simulink model "EcoSIM3_P2_C2"  (R2014b)
settings: Solver=ode1  SolverMode=SingleTasking  StartTime=0.0  StopTime=inf  FixedStep=0.01  RelTol=1e-3
PostLoadFcn:
  | %, if any(exist('dsrtsu_mdlpostloadfcn', 'file') == [2, 3, 6]), try dsrtsu_mdlpostloadfcn('Execute', bdroot); catch fprintf('Error in PostLoadFcn (dsrtsu_mdlpostloadfcn) for model "%s":\n %s\n', bdroot, lasterr); end, end,
InitFcn:
  | tic
  | %Startup_EcoSIM
undefined symbols (not defined in the file or in its folder): canChannel, Controls, DriveCycles, Driver, EM_EFF_MAP, EM_PwrLoss_MAP, EngPwr, EngSpd, EngTrq, Glbl, Plants, Power, Torque, Veh_Dynamics
libraries: canmsglib x100, canlib x87, fl_lib x78, simulink x59, nesl_utility x40, sdl_lib x17, dspsigops x5, dspswit3 x3, dspstat3 x2, commnoisgen2 x1, dspfdesign x1
(part 3 of 15)

== system EcoSIM3_P2_C2/Powertrain/Mechanical Coupler/Sensors ==
  note: Sensor Model: Place where we add Corrupter
  Ideal Rotational Motion Sensor : fl_lib/Mechanical/Mechanical Sensors/Ideal Rotational Motion Sensor  offset=0 rad
  Ideal Torque Sensor : fl_lib/Mechanical/Mechanical Sensors/Ideal Torque Sensor
  Mechanical Rotational Reference1 : fl_lib/Mechanical/Rotational Elements/Mechanical Rotational Reference
  PS-Simulink Converter : nesl_utility/PS-Simulink Converter  PhysicalDomain=network_engine_domain  SubClassName=ps_output  LeftPortType=input  RightPortType=output  PseudoPeriodic=off  Frequencies=[]  Unit=rad/s  AffineConversion=off
  PS-Simulink Converter1 : nesl_utility/PS-Simulink Converter  PhysicalDomain=network_engine_domain  SubClassName=ps_output  LeftPortType=input  RightPortType=output  PseudoPeriodic=off  Frequencies=[]  Unit=N*m  AffineConversion=off
  Terminator : Terminator
  Terminator1 : Terminator
  Shaft : PMIOPort  Port=1  Side=Left
  To_Plants : PMIOPort  Port=2  Side=Right
  wires:
  PS-Simulink Converter/1 -> Terminator/1  "MC_Speed_rad_per_s"
  PS-Simulink Converter1/1 -> Terminator1/1  "MC_Torque_Out_Nm"
  connections:
  Ideal Torque Sensor/LConn1 -- Shaft/RConn1 -- Ideal Rotational Motion Sensor/LConn1
  Ideal Rotational Motion Sensor/RConn1 -- Mechanical Rotational Reference1/LConn1
  PS-Simulink Converter/LConn1 -- Ideal Rotational Motion Sensor/RConn2
  PS-Simulink Converter1/LConn1 -- Ideal Torque Sensor/RConn2
  Ideal Torque Sensor/RConn1 -- To_Plants/RConn1

== system EcoSIM3_P2_C2/Powertrain/Soft_ECUs_IO/From_Goto ==
  Bus Creator : BusCreator  Inputs=7
  Subsystem : Subsystem
  Subsystem1 : Subsystem
  Supervisory_Wakeup_Terminated : Terminator
  tag scope: BAS_SoftECU_Receive=global, Brusa_SoftECU_Receive=global, Clutch_Trans_SoftECU_Receive=global, EM_SoftECU_Receive=global, ESS_SoftECU_Receive=global, Engine_SoftECU_Receive=global, From_ECUs=global, Supervisory_Receive=global
  wires:
  [ESS_SoftECU_Transmit] -> Bus Creator/1
  [EM_SoftECU_Transmit] -> Bus Creator/2
  [BAS_SoftECU_Transmit] -> Bus Creator/3
  [Engine_SoftECU_Transmit] -> Bus Creator/4
  Bus Creator/1 -> [From_ECUs]
  [GM_Transmit] -> Bus Creator/6
  [Clutch_Trans_SoftECU_Transmit] -> Bus Creator/5
  [From_Supervisory] -> Subsystem/1(Supervisory)
  Subsystem/1(ESS) -> [ESS_SoftECU_Receive]
  Subsystem/2(EM) -> [EM_SoftECU_Receive]
  Subsystem/3(BAS) -> [BAS_SoftECU_Receive]
  Subsystem/4(ICE) -> [Engine_SoftECU_Receive]
  Subsystem/5(Trans) -> [Clutch_Trans_SoftECU_Receive]
  Subsystem/6(Super) -> [Supervisory_Receive]
  [From_GCM] -> Subsystem1/1(From_GCM)
  Subsystem1/1(SoftECUPowerup) -> Subsystem/2(Relay Powerups)
  Subsystem1/2(MABxPowerup) -> Supervisory_Wakeup_Terminated/1
  Subsystem/7(Brusa) -> [Brusa_SoftECU_Receive]
  [Brusa_SoftECU_Transmit] -> Bus Creator/7

== system EcoSIM3_P2_C2/Powertrain/Soft_ECUs_IO/VNT Kvaser ==
  CANRx : Subsystem
  CANTx : Subsystem
  ElectricalRx : Subsystem
  ElectricalTx : Subsystem
  Spine : Subsystem
  wires:
  ElectricalRx/1(Electrical) -> Spine/1(Electrical)
  CANRx/1(CAN Out) -> Spine/2(CAN)
  Spine/1(ElectricalTx) -> ElectricalTx/1(Electrical)
  Spine/2(CANTx) -> CANTx/1(CAN)

== system EcoSIM3_P2_C2/Powertrain/Soft_ECUs_IO/VNT Vector ==
  CANRx : Subsystem
  CANTx : Subsystem
  ElectricalRx : Subsystem
  ElectricalTx : Subsystem
  Spine : Subsystem
  wires:
  ElectricalRx/1(Electrical) -> Spine/1(Electrical)
  CANRx/1(CAN Out) -> Spine/2(CAN)
  Spine/1(ElectricalTx) -> ElectricalTx/1(Electrical)
  Spine/2(CANTx) -> CANTx/1(CAN)

== system EcoSIM3_P2_C2/Powertrain/Vehicle Dynamics/Sensor ==
  Bus Creator : BusCreator  Inputs=5
  Ideal Rotational Motion Sensor{,1..3} (4 alike) : fl_lib/Mechanical/Mechanical Sensors/Ideal Rotational Motion Sensor  offset=0 rad
  Mechanical Rotational Reference{,1..3} (4 alike) : fl_lib/Mechanical/Rotational Elements/Mechanical Rotational Reference
  PS-Simulink Converter{1..2,4..5} (4 alike) : nesl_utility/PS-Simulink Converter  PhysicalDomain=network_engine_domain  SubClassName=ps_output  LeftPortType=input  RightPortType=output  PseudoPeriodic=off  Frequencies=[]  Unit=rad  AffineConversion=off
  PS-Simulink Converter3 : nesl_utility/PS-Simulink Converter  PhysicalDomain=network_engine_domain  SubClassName=ps_output  LeftPortType=input  RightPortType=output  PseudoPeriodic=off  Frequencies=[]  Unit=m/s  AffineConversion=off
  Sensor lag : Subsystem
  Sensor lag1 : Subsystem
  Sensor lag2 : Subsystem
  Sensor lag3 : Subsystem
  Sensor lag4 : Subsystem
  Vehicle_Speed : PMIOPort  Port=1  Side=Left
  FLT : PMIOPort  Port=2  Side=Left
  FRT : PMIOPort  Port=3  Side=Left
  RLT : PMIOPort  Port=4  Side=Right
  RRT : PMIOPort  Port=5  Side=Right
  Sensor_Out : Outport
  wires:
  PS-Simulink Converter3/1 -> Sensor lag/1(i)
  Sensor lag/1(o) -> Bus Creator/1  "Vehicle_Speed_meter_per_s"
  PS-Simulink Converter1/1 -> Sensor lag1/1(i)
  PS-Simulink Converter2/1 -> Sensor lag2/1(i)
  PS-Simulink Converter4/1 -> Sensor lag3/1(i)
  PS-Simulink Converter5/1 -> Sensor lag4/1(i)
  Sensor lag1/1(o) -> Bus Creator/2  "Front_Left_Tire_Angle"
  Sensor lag3/1(o) -> Bus Creator/3  "Rear_Left_Tire_Angle"
  Sensor lag2/1(o) -> Bus Creator/4  "Front_Right_Tire_Angle"
  Sensor lag4/1(o) -> Bus Creator/5  "Rear_Right_Tire_Angle"
  Bus Creator/1 -> Sensor_Out/1
  connections:
  Vehicle_Speed/RConn1 -- PS-Simulink Converter3/LConn1
  Ideal Rotational Motion Sensor/LConn1 -- FLT/RConn1
  Ideal Rotational Motion Sensor1/LConn1 -- FRT/RConn1
  Ideal Rotational Motion Sensor/RConn1 -- Mechanical Rotational Reference/LConn1
  Ideal Rotational Motion Sensor2/RConn1 -- Mechanical Rotational Reference1/LConn1
  Ideal Rotational Motion Sensor3/RConn1 -- Mechanical Rotational Reference2/LConn1
  Ideal Rotational Motion Sensor1/RConn1 -- Mechanical Rotational Reference3/LConn1
  PS-Simulink Converter1/LConn1 -- Ideal Rotational Motion Sensor/RConn3
  PS-Simulink Converter2/LConn1 -- Ideal Rotational Motion Sensor1/RConn3
  Ideal Rotational Motion Sensor2/RConn3 -- PS-Simulink Converter4/LConn1
  PS-Simulink Converter5/LConn1 -- Ideal Rotational Motion Sensor3/RConn3
  RRT/RConn1 -- Ideal Rotational Motion Sensor3/LConn1
  RLT/RConn1 -- Ideal Rotational Motion Sensor2/LConn1

== system EcoSIM3_P2_C2/Powertrain/Vehicle Dynamics/Subsystem ==
  Ideal Force Sensor : fl_lib/Mechanical/Mechanical Sensors/Ideal Force Sensor
  R : PMIOPort  Port=1  Side=Right
  C : PMIOPort  Port=2  Side=Left
  F : PMIOPort  Port=3  Side=Left
  connections:
  Ideal Force Sensor/LConn1 -- R/RConn1
  Ideal Force Sensor/RConn1 -- C/RConn1
  F/RConn1 -- Ideal Force Sensor/RConn2

== system EcoSIM3_P2_C2/RTI Data/RTI Data Store/RTI Data Store ==
  RTI Data Store : Subsystem  mask(RTI_DATA_STORE){}
      mask help:
      | RTI Data Store Block. This block is used by RTI to store internal model dependent data. Deleting this block will result in data loss.
      |
      | NEVER DELETE, COPY, OR MODIFY THIS BLOCK!
      mask Help:
      | RTI Data Store Block. This block is used by RTI to store internal model dependent data. Deleting this block will result in data loss.
      | 
      | NEVER DELETE, COPY, OR MODIFY THIS BLOCK!
      mask Display: text(0.5, 0.5, ' ', 'HorizontalAlignment', 'center');

== system EcoSIM3_P2_C2/Supervisory Controller/Driver Requested Torque/Max Torque Calculation ==
  note: at the wheels
  Gear : Inport
  Engine Speed : Inport  Port=2
  Divide2 : Product  Inputs=**
  Max Torque : Lookup_n-D  NumberOfTableDimensions=1  BreakpointsForDimension1=Plants.ICE.Mdl.Plant.Max_Trq.w  Table=Plants.ICE.Mdl.Plant.Max_Trq.Trq  InternalRulePriority=Speed  RndMeth=Simplest  InputSameDT=on
  RearGR3 : Gain  Gain=2.77
  TRAN GR2 : Lookup_n-D  NumberOfTableDimensions=1  BreakpointsForDimension1=Plants.Trans.Mdl.Plant.Gear_cmd  Table=Plants.Trans.Mdl.Plant.GR  ExtrapMethod=Clip  InternalRulePriority=Speed  RndMeth=Simplest  InputSameDT=on
  "Engine Torque " : Outport
  wires:
  TRAN GR2/1 -> Divide2/2
  Gear/1 -> TRAN GR2/1
  Engine Speed/1 -> Max Torque/1
  Divide2/1 -> "Engine Torque "/1
  Max Torque/1 -> RearGR3/1  "Engine Torque"
  RearGR3/1 -> Divide2/1

== system EcoSIM3_P2_C2/Supervisory Controller/Driver Requested Torque/Speed Calculations ==
  "Vehicle Speed m/s " : Inport
  Gear Current : Inport  Port=2
  Gain1 : Gain  Gain=2/Plants.Rear_wh.tire_diameter
  Gain2 : Gain  Gain=2.77
  Product : Product
  TRAN GR : Lookup_n-D  NumberOfTableDimensions=1  BreakpointsForDimension1=Plants.Trans.Mdl.Plant.Gear_cmd  Table=Plants.Trans.Mdl.Plant.GR  ExtrapMethod=Clip  InternalRulePriority=Speed  RndMeth=Simplest  InputSameDT=on
  Engine Speed : Outport
  "EM Speed " : Outport  Port=2
  wires:
  "Vehicle Speed m/s "/1 -> Gain1/1
  Gain2/1 -> "EM Speed "/1, Product/2
  Gain1/1 -> Gain2/1
  Product/1 -> Engine Speed/1
  Gear Current/1 -> TRAN GR/1
  TRAN GR/1 -> Product/1

== system EcoSIM3_P2_C2/Supervisory Controller/Functional Safety1/Functional Safety Algorithm ==
  Torque Requests : Inport
  ECU/Sensor Signals : Inport  Port=2
  Fault Detection (Team Developed) : Subsystem
  Fault Management : Subsystem
  Fault Mitigation : Subsystem
  Torque Limits : Outport
  Fault Code : Outport  Port=2
  wires:
  Torque Requests/1 -> Fault Detection (Team Developed)/1(Torque Requests)
  ECU/Sensor Signals/1 -> Fault Detection (Team Developed)/2(ECU/Sensor Signals), Fault Management/2(ECU/Sensor Signals)
  Fault Mitigation/1(Torque Limits) -> Torque Limits/1
  Fault Management/1(Fault Code) -> Fault Mitigation/1(Fault Code), Fault Code/1
  Fault Detection (Team Developed)/1(Team Dev Fault Signals) -> Fault Management/1(Team Dev Fault Signals)

== system EcoSIM3_P2_C2/Supervisory Controller/Input Conditioning/Alpha Conditioning ==
  Raw Alpha_V : Inport
  Add : Sum
  Bus Selector : BusSelector  OutputSignals=GM_Transmit.GM_Electrical_Out.Alpha_Low,GM_Transmit.GM_Electrical_Out.Alpha_High
  Constant : Constant  Value=0.4
  Constant1 : Constant  Value=0.8
  Output Scaling5 : Gain  Gain=50
  Output Scaling6 : Gain  Gain=25
  Output Scaling7 : Gain  Gain=0.5
  Sum4 : Sum  Inputs=-+|
  Sum5 : Sum  Inputs=|+-
  Alpha Percent : Outport
  wires:
  Constant1/1 -> Sum5/2
  Sum5/1 -> Output Scaling6/1
  Output Scaling5/1 -> Add/1
  Output Scaling7/1 -> Alpha Percent/1  "Alpha_percent"
  Bus Selector/1 -> Sum4/2  "<Alpha_Low>"
  Output Scaling6/1 -> Add/2
  Constant/1 -> Sum4/1
  Add/1 -> Output Scaling7/1
  Sum4/1 -> Output Scaling5/1
  Bus Selector/2 -> Sum5/1  "<Alpha_High>"
  Raw Alpha_V/1 -> Bus Selector/1

== system EcoSIM3_P2_C2/Supervisory Controller/Input Conditioning/Velocity Conditioning ==
  Raw Ticks : Inport
  Bus Creator : BusCreator  Inputs=2
  Bus Selector1 : BusSelector  OutputSignals=GM_Transmit.GMLAN_CAN_Out.PPEI_Vehicle_Speed_and_Distance.VehSpdAvgDrvn,GM_Transmit.GMLAN_CAN_Out.PPEI_Driven_Whl_Rotational_Stat.WRSLDWhlDistPlsCntr,GM_Transmit.GMLAN_CAN_Out.PPEI_Driven_Whl_Rotational_Stat.WRSRDWhlDistPlsCntr,GM_Transmit.GMLAN_CAN_Out.PPEI_NonDrivn_Whl_Rotationl_Stat.WRSLNDWhlDistPCntr,GM_Transmit.GMLAN_CAN_Out.PPEI_NonDrivn_Whl_Rotationl_Stat.WRSRNDWhlDistPCntr
  Gain : Gain  Gain=1/3.6
  Mean : dspstat3/Mean  run=off  reset_popup=None  InputProcessing=Columns as channels (frame based)  directionMode=Each column  dimension=1  treatSBRowAsCol=on  roiEnable=off  roiType=Rectangles  roiPortion=Entire ROI  roiOutput=Individual statistics for each ROI  roiFlag=off  outputDataTypeStr=Inherit: Same as accumulator  outputLastDataTypeStr=Inherit: Same as accumulator  outputMin=[]  outputMax=[]  roundingMode=Floor  overflowMode=off
  Mux : Mux
  Subsystem : Subsystem
  Subsystem1 : Subsystem
  Subsystem2 : Subsystem
  Subsystem3 : Subsystem
  Velocity Processed : Outport
  wires:
  Bus Selector1/5 -> Subsystem3/1(In1)  "<WRSRNDWhlDistPCntr>"
  Bus Selector1/4 -> Subsystem2/1(In1)  "<WRSLNDWhlDistPCntr>"
  Raw Ticks/1 -> Bus Selector1/1
  Bus Selector1/1 -> Gain/1  "<VehSpdAvgDrvn>"
  Bus Selector1/3 -> Subsystem1/1(In1)  "<WRSRDWhlDistPlsCntr>"
  Bus Creator/1 -> Velocity Processed/1  "Vehicle_speed"
  Mean/1 -> Bus Creator/2  "Processed_Speed_m_per_sec"
  Gain/1 -> Bus Creator/1  "Vehicle_Speed_meter_per_s"
  Bus Selector1/2 -> Subsystem/1(In1)  "<WRSLDWhlDistPlsCntr>"
  Subsystem2/1(Speed_LND) -> Mux/3
  Subsystem1/1(Speed_RD) -> Mux/2
  Subsystem/1(Speed_LD) -> Mux/1
  Subsystem3/1(Speed_RND) -> Mux/4
  Mux/1 -> Mean/1

== system EcoSIM3_P2_C2/Supervisory Controller/Mode Operation/Accessory ==
  "Supervisory " : Inport
  Enable : EnablePort  StatesWhenEnabling=reset
  BAS_Signals : Subsystem
  Bus Creator2 : BusCreator  Inputs=8
  Constant1 : Constant  Value=0
  DC/DC Enabled : Subsystem
  ESS_Messages : Subsystem
  Engine Messages : Subsystem
  Signal Conversion : SignalConversion
  TM Messages : Subsystem
  Trans_Messages : Subsystem
  Output : Outport
  wires:
  Signal Conversion/1 -> Output/1  "HSC_Output"
  Engine Messages/1(Out1) -> Bus Creator2/5
  ESS_Messages/1(Out1) -> Bus Creator2/2  "ESS_Signals_A123"
  Trans_Messages/1(Out1) -> Bus Creator2/6  "Trans_Receive"
  BAS_Signals/1(Out1) -> Bus Creator2/4  "BAS_SoftECU_Receive"
  "Supervisory "/1 -> Bus Creator2/7  "Supervisory"
  Bus Creator2/1 -> Signal Conversion/1  "HSC_Output"
  DC/DC Enabled/1(Out1) -> Bus Creator2/8
  TM Messages/1(Out1) -> Bus Creator2/3
  Constant1/1 -> Bus Creator2/1  "Vehicle_Ready"

== system EcoSIM3_P2_C2/Supervisory Controller/Mode Operation/Charging ==
  From CAN : Inport
  "Supervisory " : Inport  Port=2
  Enable : EnablePort  StatesWhenEnabling=reset
  BAS_Signals : Subsystem
  Bus Creator2 : BusCreator  Inputs=8
  Constant2 : Constant  Value=0
  DC/DC Enabled : Subsystem
  EM_Signals : Subsystem
  ESS_Messages : Subsystem
  Engine Messages : Subsystem
  Signal Conversion : SignalConversion
  Trans_Messages : Subsystem
  Output : Outport
  wires:
  Signal Conversion/1 -> Output/1  "HSC_Output"
  Engine Messages/1(Out1) -> Bus Creator2/5
  ESS_Messages/1(Out1) -> Bus Creator2/2  "ESS_Signals_A123"
  Trans_Messages/1(Out1) -> Bus Creator2/6  "Trans_Receive"
  BAS_Signals/1(Out1) -> Bus Creator2/4  "BAS_SoftECU_Receive"
  From CAN/1 -> ESS_Messages/1(From CAN)
  "Supervisory "/1 -> Bus Creator2/7  "Supervisory"
  Bus Creator2/1 -> Signal Conversion/1  "HSC_Output"
  EM_Signals/1(Out1) -> Bus Creator2/3
  DC/DC Enabled/1(Out1) -> Bus Creator2/8
  Constant2/1 -> Bus Creator2/1  "Vehicle_Ready"

== system EcoSIM3_P2_C2/Supervisory Controller/Mode Operation/EV ==
  "Supervisory " : Inport
  CAN : Inport  Port=2
  Enable : EnablePort  StatesWhenEnabling=reset
  BAS_Signals : Subsystem
  Bus Creator1 : BusCreator  Inputs=8
  Bus Creator2 : BusCreator  Inputs=3
  Bus Selector : BusSelector  OutputSignals=Driver Torque Request
  Bus Selector1 : BusSelector  OutputSignals=EM_Transmit.EM_CAN_Out.M165_Motor_Position_Info.Motor_Speed,EM_Transmit.EM_CAN_Out.M162_Temperature_Set_3.Motor_Temperature
  Constant1 : Constant  Value=0
  Constant2 : Constant
  Constant4 : Constant
  Constant5 : Constant  Value=0
  DC/DC Enabled : Subsystem
  EM Max Torque1 : Lookup_n-D  NumberOfTableDimensions=1  BreakpointsForDimension1=Plants.EM.Mdl.Plant.max_min_RPM  BreakpointsForDimension2=[25,70]  Table=[Plants.EM.Mdl.Plant.T_max_Peak]  InternalRulePriority=Speed  RndMeth=Simplest  InputSameDT=on
  ESS_Messages : Subsystem
  Engine Messages : Subsystem
  Gain : Gain  Gain=1/(2.77*2.77)
  Saturation Dynamic : simulink/Discontinuities/Saturation Dynamic  OutMin=[]  OutMax=[]  OutDataTypeStr=Inherit: Same as second input  OutDataType=fixdt(1, 16)  OutScaling=2^-10  DoSatur=off
  Signal Conversion : SignalConversion
  Trans_Messages : Subsystem
  Output : Outport
  wires:
  Signal Conversion/1 -> Output/1  "HSC_Output"
  Engine Messages/1(Out1) -> Bus Creator1/5
  ESS_Messages/1(Out1) -> Bus Creator1/2  "ESS_Signals_A123"
  Bus Creator2/1 -> Bus Creator1/3  "EM_Messages_Rhinehart"
  Gain/1 -> Saturation Dynamic/2  "Torque_Command"
  Constant1/1 -> Bus Creator2/3  "Rotation_Direction"
  Constant2/1 -> Bus Creator2/1  "Inverter_Enable"
  Trans_Messages/1(Out1) -> Bus Creator1/6  "Trans_Receive"
  BAS_Signals/1(Out1) -> Bus Creator1/4  "BAS_SoftECU_Receive"
  "Supervisory "/1 -> Bus Creator1/7, Bus Selector/1  "Supervisory"
  Bus Creator1/1 -> Signal Conversion/1  "HSC_Output"
  Bus Selector/1 -> Gain/1  "<Driver Torque Request>"
  Constant4/1 -> Bus Creator1/1  "Vehicle_Ready"
  DC/DC Enabled/1(Out1) -> Bus Creator1/8
  Saturation Dynamic/1 -> Bus Creator2/2  "Torque_Command"
  Constant5/1 -> Saturation Dynamic/3
  CAN/1 -> Bus Selector1/1
  Bus Selector1/1 -> EM Max Torque1/1  "<Motor_Speed>"
  Bus Selector1/2 -> ?  "<Motor_Temperature>"
  EM Max Torque1/1 -> Saturation Dynamic/1

== system EcoSIM3_P2_C2/Supervisory Controller/Mode Operation/Engine Only  ==
  note: this will end up being engine idle in the vehicle
  "Supervisory " : Inport
  From CAN : Inport  Port=2
  Enable : EnablePort  StatesWhenEnabling=reset
  BAS_Signals : Subsystem
  Bus Creator1 : BusCreator  Inputs=8
  Bus Creator6 : BusCreator  Inputs=2
  Constant1 : Constant
  Constant2 : Constant  Value=0
  Constant4 : Constant
  DC/DC Enabled : Subsystem
  ESS_Messages : Subsystem
  Engine Messages : Subsystem
  Signal Conversion : SignalConversion
  Subsystem : Subsystem
  Supervisory 1 : InportShadow
  TM Messages : Subsystem
  Terminator : Terminator
  Terminator1 : Terminator
  "Output " : Outport
  wires:
  Signal Conversion/1 -> "Output "/1  "HSC_Output"
  ESS_Messages/1(Out1) -> Bus Creator1/2  "ESS_Signals_A123"
  Bus Creator6/1 -> Bus Creator1/6  "Trans_Receive"
  BAS_Signals/1(Out1) -> Bus Creator1/4  "BAS_SoftECU_Receive"
  Constant2/1 -> Bus Creator6/1  "Shift_Request"
  Subsystem/3("Gear Requested ") -> Terminator1/1  "Gear_Request"
  "Supervisory "/1 -> Bus Creator1/7, Subsystem/2(Supervisory)  "Supervisory"
  Bus Creator1/1 -> Signal Conversion/1  "HSC_Output"
  From CAN/1 -> Subsystem/1(From CAN)
  Subsystem/2(Shift Requested) -> Terminator/1
  Constant1/1 -> Bus Creator6/2  "Gear_Request"
  Constant4/1 -> Bus Creator1/1  "Vehicle_Ready"
  DC/DC Enabled/1(Out1) -> Bus Creator1/8
  TM Messages/1(Out1) -> Bus Creator1/3
  Engine Messages/1(Out1) -> Bus Creator1/5
  Supervisory 1/1 -> TM Messages/1(In1)  "Supervisory"

== system EcoSIM3_P2_C2/Supervisory Controller/Mode Operation/Engine Start  ==
  "Supervisory " : Inport
  "CAN In " : Inport  Port=2
  Enable : EnablePort  StatesWhenEnabling=reset
  1-D Lookup Table : Lookup_n-D  NumberOfTableDimensions=1  BreakpointsForDimension1=[0 2699 2700 3000 3239 3240]  Table=[11.11 11.11 8 5.5 5.5 0]  InternalRulePriority=Speed  RndMeth=Simplest  InputSameDT=on
  Bus Creator1 : BusCreator  Inputs=8
  Bus Creator2 : BusCreator  Inputs=3
  Bus Creator4 : BusCreator  Inputs=3
  Bus Selector : BusSelector  OutputSignals=BAS_Transmit.BAS_CAN_Out.Status_1.BAS_Speed_rad_per_s
  Compare To Constant : simulink/Logic and Bit Operations/Compare To Constant  relop=>  const=900  OutDataTypeStr=boolean
  Constant1 : Constant  Value=0
  Constant3 : Constant  Value=0
  Constant4 : Constant
  Constant5 : Constant
  Constant6 : Constant
  Convert to Engine Speed : Gain  Gain=1/2.7
  DC/DC Enabled : Subsystem
  Data Type Conversion : DataTypeConversion  OutDataTypeStr=double
  ESS_Messages : Subsystem
  Sample and Hold : dspsigops/Sample and Hold  trig=Rising edge  initCond=0  latchinput=off
  Signal Conversion : SignalConversion
  Supervisory 1 : InportShadow
  TM Messages : Subsystem
  Trans Messages : Subsystem
  rad/sec to RPM : Gain  Gain=9.54929659643
  rad/sec to RPM1 : Gain  Gain=1.1
  "Output " : Outport
  wires:
  Signal Conversion/1 -> "Output "/1  "HSC_Output"
  ESS_Messages/1(Out1) -> Bus Creator1/2  "ESS_Signals_A123"
  "Supervisory "/1 -> Bus Creator1/7  "Supervisory"
  Bus Creator1/1 -> Signal Conversion/1  "HSC_Output"
  Constant5/1 -> Bus Creator1/1  "Vehicle_Ready"
  DC/DC Enabled/1(Out1) -> Bus Creator1/8
  TM Messages/1(Out1) -> Bus Creator1/3
  Constant6/1 -> Bus Creator4/3  "BAS_Mode_Request"
  Bus Creator4/1 -> Bus Creator1/4  "BAS_SoftECU_Receive"
  Trans Messages/1(Out1) -> Bus Creator1/6
  Supervisory 1/1 -> TM Messages/1(In1)  "Supervisory"
  Constant3/1 -> Bus Creator2/1  "ICE_Torque_Request_Nm"
  1-D Lookup Table/1 -> rad/sec to RPM1/1  "BAS_Torque_Request_Nm"
  Constant1/1 -> Bus Creator4/2  "BAS_Speed_Request"
  Constant4/1 -> Bus Creator2/2  "Engine_On"
  "CAN In "/1 -> Bus Selector/1
  Bus Selector/1 -> rad/sec to RPM/1  "<BAS_Speed_rad_per_s>"
  rad/sec to RPM/1 -> Convert to Engine Speed/1, 1-D Lookup Table/1  "BAS_Speed_RPM"
  Bus Creator2/1 -> Bus Creator1/5  "ICE_Request"
  Compare To Constant/1 -> Data Type Conversion/1
  Convert to Engine Speed/1 -> Compare To Constant/1
  Data Type Conversion/1 -> Sample and Hold/Trigger, Sample and Hold/1  "Engine_Run"
  Sample and Hold/1 -> Bus Creator2/3  "Engine_Run"
  rad/sec to RPM1/1 -> Bus Creator4/1  "BAS_Torque_Request_Nm"

== system EcoSIM3_P2_C2/Supervisory Controller/Mode Operation/Limited EV ==
  "Supervisory " : Inport
  CAN : Inport  Port=2
  Enable : EnablePort  StatesWhenEnabling=reset
  BAS_Signals : Subsystem
  Bus Creator3 : BusCreator  Inputs=8
  Bus Creator4 : BusCreator  Inputs=3
  Bus Selector : BusSelector  OutputSignals=Driver Torque Request
  Bus Selector1 : BusSelector  OutputSignals=EM_Transmit.EM_CAN_Out.M162_Temperature_Set_3.Motor_Temperature,ESS_Transmit.ESS_CAN_Out.BCM_Data1.bcm_cell_tmax,EM_Transmit
  Constant1 : Constant
  Constant2 : Constant  Value=0
  Constant4 : Constant
  DC/DC Enabled : Subsystem
  ESS_Messages : Subsystem
  Engine Messages : Subsystem
  Gain1 : Gain  Gain=1/(2.77*2.77)
  "Inverter Temp Selection " : Subsystem
  Signal Conversion : SignalConversion
  Temperature Limiting : Subsystem
  Trans_Messages : Subsystem
  Output : Outport
  wires:
  Signal Conversion/1 -> Output/1  "HSC_Output"
  ESS_Messages/1(Out1) -> Bus Creator3/2  "ESS_Signals_A123"
  Bus Creator4/1 -> Bus Creator3/3  "EM_Messages_Rhinehart"
  Bus Selector/1 -> Gain1/1  "<Driver Torque Request>"
  Constant2/1 -> Bus Creator4/3  "Rotation_Direction"
  Constant4/1 -> Bus Creator4/1  "Inverter_Enable"
  Trans_Messages/1(Out1) -> Bus Creator3/6  "Trans_Receive"
  BAS_Signals/1(Out1) -> Bus Creator3/4  "BAS_SoftECU_Receive"
  "Supervisory "/1 -> Bus Creator3/7, Bus Selector/1  "Supervisory"
  Bus Creator3/1 -> Signal Conversion/1  "HSC_Output"
  Constant1/1 -> Bus Creator3/1  "Vehicle_Ready"
  DC/DC Enabled/1(Out1) -> Bus Creator3/8
  Gain1/1 -> Temperature Limiting/1(Torque Request)  "Torque_Command"
  Bus Selector1/1 -> Temperature Limiting/2("Motor Temperature ")  "<Motor_Temperature>"
  "Inverter Temp Selection "/1(Out1) -> Temperature Limiting/4("Inverter Temperature ")
  CAN/1 -> Bus Selector1/1
  Temperature Limiting/1(Torque Command) -> Bus Creator4/2  "Torque_Command"
  Bus Selector1/2 -> Temperature Limiting/3("Battery Temperature ")  "<bcm_cell_tmax>"
  Engine Messages/1(Out1) -> Bus Creator3/5
  Bus Selector1/3 -> "Inverter Temp Selection "/1(In1)  "<EM_Transmit>"

== system EcoSIM3_P2_C2/Supervisory Controller/Mode Operation/Series ==
  "Supervisory " : Inport
  From CAN : Inport  Port=2
  Enable : EnablePort  StatesWhenEnabling=reset
  Bus Creator1 : BusCreator  Inputs=8
  Bus Creator2 : BusCreator  Inputs=3
  Bus Creator4 : BusCreator  Inputs=3
  Bus Creator5 : BusCreator  Inputs=3
  Bus Selector : BusSelector  OutputSignals=Driver Torque Request
  Constant1 : Constant  Value=2
  Constant{2,5,7..8} (4 alike) : Constant
  Constant3 : Constant  Value=0
  Constant4 : Constant  Value=0
  DC/DC Enabled : Subsystem
  ESS_Messages : Subsystem
  Gain : Gain
  Gain1 : Gain  Gain=1/(2.77*2.77)
  "Series Torque Determination " : Subsystem
  Signal Conversion : SignalConversion
  Supervisory 1 : InportShadow
  Trans_Messages : Subsystem
  "Output " : Outport
  wires:
  Bus Creator1/1 -> Signal Conversion/1  "HSC_Output"
  "Supervisory "/1 -> Bus Creator1/7  "Supervisory"
  Bus Selector/1 -> Gain1/1  "<Driver Torque Request>"
  Supervisory 1/1 -> Bus Selector/1  "Supervisory"
  Constant5/1 -> Bus Creator5/1  "Inverter_Enable"
  Constant3/1 -> Bus Creator5/3  "Rotation_Direction"
  Bus Creator5/1 -> Bus Creator1/3  "EM_Messages_Rhinehart"
  ESS_Messages/1(Out1) -> Bus Creator1/2  "ESS_Signals_A123"
  Signal Conversion/1 -> "Output "/1  "HSC_Output"
  Trans_Messages/1(Out1) -> Bus Creator1/6  "Trans_Receive"
  Bus Creator4/1 -> Bus Creator1/4  "BAS_SoftECU_Receive"
  Constant1/1 -> Bus Creator4/3  "BAS_Mode_Request"
  DC/DC Enabled/1(Out1) -> Bus Creator1/8
  Constant2/1 -> Bus Creator1/1  "Vehicle_Ready"
  Gain1/1 -> Bus Creator5/2  "Torque_Command"
  "Series Torque Determination "/2(Engine Torque) -> Gain/1
  "Series Torque Determination "/1(BAS Speed) -> Bus Creator4/2  "BAS_Speed_Request"
  Constant4/1 -> Bus Creator4/1  "BAS_Torque_Request_Nm"
  From CAN/1 -> "Series Torque Determination "/1(Battery SOC)
  Gain/1 -> Bus Creator2/1  "ICE_Torque_Request_Nm"
  Constant7/1 -> Bus Creator2/2  "Engine_On"
  Constant8/1 -> Bus Creator2/3  "Engine_Run"
  Bus Creator2/1 -> Bus Creator1/5  "ICE_Request"

== system EcoSIM3_P2_C2/Supervisory Controller/Mode Operation/Shutdown ==
  From CAN : Inport
  "Supervisory " : Inport  Port=2
  Enable : EnablePort  StatesWhenEnabling=reset
  BAS_Signals : Subsystem
  Bus Creator2 : BusCreator  Inputs=8
  Bus Creator3 : BusCreator  Inputs=3
  Bus Selector : BusSelector  OutputSignals=EM_Transmit.EM_CAN_Out.M170_Internal_States.Inverter_Enable_Lockout
  Constant3 : Constant  Value=0
  Constant6 : Constant  Value=0
  DC/DC Disabled : Subsystem
  EM Handshake : Stateflow chart  TreatAsAtomicUnit=on
  Engine Messages : Subsystem
  Shutdown : Subsystem
  Shutdown Complete : Subsystem
  Signal Conversion : SignalConversion
  Trans_Messages : Subsystem
  Output : Outport
  wires:
  Signal Conversion/1 -> Output/1  "HSC_Output"
  Engine Messages/1(Out1) -> Bus Creator2/5
  Shutdown/1(Out1) -> Shutdown Complete/1(In1), Bus Creator2/2
  Bus Creator3/1 -> Bus Creator2/3  "EM_Messages_Rhinehart"
  Constant6/1 -> Bus Creator3/2  "Torque_Command"
  Constant3/1 -> Bus Creator3/3  "Rotation_Direction"
  EM Handshake/1(Inverter_Enable) -> Shutdown Complete/2(In2), Bus Creator3/1  "Inverter_Enable"
  Trans_Messages/1(Out1) -> Bus Creator2/6  "Trans_Receive"
  BAS_Signals/1(Out1) -> Bus Creator2/4  "BAS_SoftECU_Receive"
  From CAN/1 -> Shutdown/1(In1), Bus Selector/1
  "Supervisory "/1 -> Bus Creator2/7  "Supervisory"
  Bus Selector/1 -> EM Handshake/1(Inverter_Enable_Lockout)  "<Inverter_Enable_Lockout>"
  Bus Creator2/1 -> Signal Conversion/1  "HSC_Output"
  DC/DC Disabled/1(Out1) -> Bus Creator2/8
  Shutdown Complete/1(Out1) -> Bus Creator2/1  "Vehicle_Ready"

== system EcoSIM3_P2_C2/Supervisory Controller/Mode Operation/Startup ==
  From CAN : Inport
  "Supervisory " : Inport  Port=2
  Enable : EnablePort  StatesWhenEnabling=reset
  BAS Start up : Subsystem
  "Battery Start Up " : Subsystem
  Bus Creator1 : BusCreator  Inputs=8
  Bus Selector : BusSelector  OutputSignals=ESS_Transmit.ESS_CAN_Out.BCM_Status.bcm_mainc_stat
  Bus Selector1 : BusSelector  OutputSignals=Inverter_Enable
  Bus Selector2 : BusSelector  OutputSignals=BAS_Mode_Request
  DC/DC Enabled : Subsystem
  EM Start up : Subsystem
  Engine Messages : Subsystem
  Signal Conversion : SignalConversion
  "Start up overide " : Subsystem
  To Workspace : ToWorkspace  VariableName=StartComplete  SaveFormat=Structure With Time  SampleTime=-1
  To Workspace1 : ToWorkspace  VariableName=bcm_mainc_stat  SaveFormat=Structure With Time  SampleTime=-1
  To Workspace2 : ToWorkspace  VariableName=Inverter_enable  SaveFormat=Structure With Time  SampleTime=-1
  To Workspace3 : ToWorkspace  VariableName=BAS_Enabled  SaveFormat=Structure With Time  SampleTime=-1
  To Workspace4 : ToWorkspace  VariableName=VehReady2  SaveFormat=Structure With Time  SampleTime=-1
  Trans_Messages : Subsystem
  Vehicle Ready : Stateflow chart  TreatAsAtomicUnit=on
  "Vehicle Start Up " : Subsystem
  Output : Outport
  wires:
  Bus Creator1/1 -> Signal Conversion/1
  BAS Start up/1(Out1) -> Bus Selector2/1, Bus Creator1/4  "BAS_SoftECU_Receive"
  Trans_Messages/1(Out1) -> Bus Creator1/6  "Trans_Receive"
  "Battery Start Up "/1(Out1) -> Bus Creator1/2
  EM Start up/1(Out1) -> Bus Selector1/1, Bus Creator1/3
  Bus Selector/1 -> To Workspace1/1, Vehicle Ready/2(bcm_mainc_stat)  "<bcm_mainc_stat>"
  Bus Selector1/1 -> Vehicle Ready/3(Inverter_Enable), To Workspace2/1  "<Inverter_Enable>"
  Bus Selector2/1 -> To Workspace3/1, Vehicle Ready/4(BAS_Mode_Request)  "<BAS_Mode_Request>"
  Vehicle Ready/1(Vehicle_Ready) -> To Workspace4/1, Bus Creator1/1  "Vehicle_Ready"
  "Supervisory "/1 -> Bus Creator1/7  "Supervisory"
  Signal Conversion/1 -> Output/1  "HSC_Output"
  "Vehicle Start Up "/1(Start) -> Vehicle Ready/1(Startup_Complete), To Workspace/1
  From CAN/1 -> "Start up overide "/1(In1), BAS Start up/1(In1), EM Start up/1(In1), "Battery Start Up "/1(CAN), Bus Selector/1
  DC/DC Enabled/1(Out1) -> Bus Creator1/8
  Engine Messages/1(Out1) -> Bus Creator1/5
  "Start up overide "/1(Out1) -> "Vehicle Start Up "/1(In1)

== system EcoSIM3_P2_C2/Supervisory Controller/Mode Selection /Limp Home Mode Selection   ==
  "Mode Requested  " : Inport
  "Fault Code " : Inport  Port=2
  Chart : Stateflow chart  TreatAsAtomicUnit=on
  Data Type Conversion : DataTypeConversion  OutDataTypeStr=double
  Fault Counter : Subsystem
  Sample and Hold : dspsigops/Sample and Hold  trig=Rising edge  initCond=0  latchinput=off
  Scope : Scope
      settings: YMin=1.625  YMax=5.375  SaveName=ScopeData6
  Switch : Switch  Criteria=u2 > Threshold  OutDataTypeStr=Inherit: Inherit via back propagation
  Transport Delay : TransportDelay  DelayTime=.1
  Vehicle Mode : Outport
  wires:
  "Mode Requested  "/1 -> Switch/3
  Switch/1 -> Vehicle Mode/1
  Chart/1(VEH_Mode) -> Scope/1, Switch/1
  "Fault Code "/1 -> Data Type Conversion/1
  Fault Counter/1(Fault_Code) -> Chart/1(Fault_Code)
  Sample and Hold/1 -> Switch/2
  Transport Delay/1 -> Fault Counter/1(In1), Sample and Hold/1, Sample and Hold/Trigger
  Data Type Conversion/1 -> Transport Delay/1

== system EcoSIM3_P2_C2/Supervisory Controller/PRNDL/Determine Gear ==
  From CAN : Inport
  HSC Inputs : Inport  Port=2
  Bus Selector : BusSelector  OutputSignals=GM_Transmit.GM_Electrical_Out.PRNDL,ESS_Transmit.ESS_CAN_Out.BCM_Status.bcm_epo,GM_Transmit.GMLAN_CAN_Out.PPEI_Platform_General_Status.SysPwrMd,ESS_Transmit.ESS_CAN_Out.BCM_Status.bcm_on_plug
  Bus Selector1 : BusSelector  OutputSignals=Vehicle_Ready
  Compare To Constant : simulink/Logic and Bit Operations/Compare To Constant  relop=<  const=2  OutDataTypeStr=boolean  ZeroCross=off
  Data Type Conversion : DataTypeConversion
  Display{,1..5} (6 alike) : Display
  Logical Operator : Logic  Operator=OR  Inputs=4  AllPortsSameDT=off  OutDataTypeStr=boolean
  Logical Operator1 : Logic  Operator=NOT  AllPortsSameDT=off  OutDataTypeStr=boolean
  Subsystem : Subsystem
  Truth Table : Truth Table  TreatAsAtomicUnit=on
  Gear : Outport
  wires:
  Bus Selector/1 -> Display/1, Subsystem/1(PRNDL Position), Truth Table/1(PRNDL)  "<PRNDL>"
  From CAN/1 -> Bus Selector/1
  Logical Operator/1 -> Truth Table/3(Force_Park)
  Logical Operator1/1 -> Data Type Conversion/1
  Data Type Conversion/1 -> Logical Operator/4
  Compare To Constant/1 -> Logical Operator/2
  Bus Selector/4 -> Display3/1, Logical Operator/3  "<bcm_on_plug>"
  Bus Selector1/1 -> Display4/1, Logical Operator1/1  "<Vehicle_Ready>"
  Truth Table/1(y) -> Display5/1, Gear/1
  Bus Selector/3 -> Display2/1, Compare To Constant/1  "<SysPwrMd>"
  HSC Inputs/1 -> Bus Selector1/1
  Bus Selector/2 -> Display1/1, Subsystem/2(bcm_epo)  "<bcm_epo>"
  Subsystem/1(Force Neutral) -> Truth Table/2(Force_Neutral)
  Subsystem/2(Force Park) -> Logical Operator/1

== system EcoSIM3_P2_C2/Supervisory Controller/PRNDL/Determine Gear1 ==
  In1 : Inport
  In2 : Inport  Port=2
  Bus Selector : BusSelector  OutputSignals=GM_Transmit.GM_Electrical_Out.PRNDL,ESS_Transmit.ESS_CAN_Out.BCM_Status.bcm_epo,GM_Transmit.GM_Electrical_Out.Key_State
  Bus Selector1 : BusSelector  OutputSignals=Vehicle_Ready
  Compare To Constant : simulink/Logic and Bit Operations/Compare To Constant  relop=<  const=2  OutDataTypeStr=boolean  ZeroCross=off
  Data Type Conversion : DataTypeConversion
  Logical Operator : Logic  Operator=OR  Inputs=4  AllPortsSameDT=off  OutDataTypeStr=boolean
  Logical Operator1 : Logic  Operator=NOT  AllPortsSameDT=off  OutDataTypeStr=boolean
  Truth Table : Truth Table  TreatAsAtomicUnit=on
  bcm_on_plug : Constant  Value=0
  Gear : Outport
  wires:
  Bus Selector/1 -> Truth Table/1(PRNDL)  "<PRNDL>"
  In1/1 -> Bus Selector/1
  Truth Table/1(y) -> Gear/1
  Logical Operator/1 -> Truth Table/2(Force_Neutral)
  Bus Selector/3 -> Compare To Constant/1  "<Key_State>"
  In2/1 -> Bus Selector1/1
  Logical Operator1/1 -> Data Type Conversion/1
  Data Type Conversion/1 -> Logical Operator/3
  Compare To Constant/1 -> Logical Operator/4
  bcm_on_plug/1 -> Logical Operator/1
  Bus Selector/2 -> Logical Operator/2  "<bcm_epo>"
  Bus Selector1/1 -> Logical Operator1/1  "<Vehicle_Ready>"

== system EcoSIM3_P2_C2/Supervisory Controller/PRNDL/Drive ==
  In1 : Inport
  Enable : EnablePort
  Bus Creator : BusCreator  Inputs=6
  Bus Creator1 : BusCreator  Inputs=3
  Bus Creator2 : BusCreator  Inputs=3
  Bus Creator4 : BusCreator  Inputs=3
  Bus Selector : BusSelector  OutputSignals=ESS_Signals_A123,EM_Messages_Rhinehart.Inverter_Enable,EM_Messages_Rhinehart.Torque_Command,EM_Messages_Rhinehart.Rotation_Direction,BAS_SoftECU_Receive.BAS_Torque_Request_Nm,BAS_SoftECU_Receive.BAS_Speed_Request,BAS_SoftECU_Receive.BAS_Mode_Request,ICE_Request.ICE_Torque_Request_Nm,ICE_Request.Engine_On,ICE_Request.Engine_Run,Trans_Receive,Supervisory
  Check BAS Limits : Subsystem
  Check EM Limits : Subsystem
  Check Engine Limits : Subsystem
  HSC_Out : Outport
  wires:
  Bus Creator/1 -> HSC_Out/1  "HSC_Out"
  In1/1 -> Bus Selector/1
  Bus Selector/1 -> Bus Creator/1  "<ESS_Signals_A123>"
  Bus Selector/2 -> Bus Creator1/1  "<Inverter_Enable>"
  Bus Selector/3 -> Check EM Limits/1(In1)  "<Torque_Command>"
  Bus Selector/4 -> Bus Creator1/3  "<Rotation_Direction>"
  Bus Creator1/1 -> Bus Creator/2  "EM_Messages_Rhinehart"
  Bus Selector/5 -> Check BAS Limits/1(In1)  "<BAS_Torque_Request_Nm>"
  Bus Selector/7 -> Bus Creator2/3  "<BAS_Mode_Request>"
  Bus Creator2/1 -> Bus Creator/3  "BAS_SoftECU_Receive"
  Bus Selector/8 -> Check Engine Limits/1(In1)  "<ICE_Torque_Request_Nm>"
  Bus Selector/11 -> Bus Creator/5  "<Trans_Receive>"
  Check BAS Limits/1(Out1) -> Bus Creator2/1  "BAS_Torque_Request_Nm"
  Check EM Limits/1(Out1) -> Bus Creator1/2  "Torque_Command"
  Bus Selector/12 -> Bus Creator/6  "<Supervisory>"
  Bus Selector/6 -> Bus Creator2/2  "<BAS_Speed_Request>"
  Bus Creator4/1 -> Bus Creator/4  "Engine_Messages"
  Bus Selector/9 -> Bus Creator4/2  "<Engine_On>"
  Bus Selector/10 -> Bus Creator4/3  "<Engine_Run>"
  Check Engine Limits/1(Out1) -> Bus Creator4/1  "ICE_Torque_Request_Nm"

== system EcoSIM3_P2_C2/Supervisory Controller/PRNDL/Neutral  ==
  Treq : Inport
  Enable : EnablePort
  Bus Creator1 : BusCreator  Inputs=6
  Bus Creator2 : BusCreator  Inputs=3
  Bus Creator3 : BusCreator  Inputs=3
  Bus Creator4 : BusCreator  Inputs=3
  Bus Selector : BusSelector  OutputSignals=ESS_Signals_A123,EM_Messages_Rhinehart.Inverter_Enable,EM_Messages_Rhinehart.Torque_Command,EM_Messages_Rhinehart.Rotation_Direction,BAS_SoftECU_Receive.BAS_Speed_Request,BAS_SoftECU_Receive.BAS_Mode_Request,ICE_Request.ICE_Torque_Request_Nm,ICE_Request.Engine_On,ICE_Request.Engine_Run,Trans_Receive,Supervisory
  ICE{2..6} (5 alike) : Constant  Value=0
  Terminator{,1..3} (4 alike) : Terminator
  "HSC_Out " : Outport
  wires:
  Bus Creator1/1 -> "HSC_Out "/1  "HSC_Out"
  Treq/1 -> Bus Selector/1
  Bus Selector/1 -> Bus Creator1/1  "<ESS_Signals_A123>"
  Bus Selector/2 -> Bus Creator2/1  "<Inverter_Enable>"
  Bus Selector/3 -> Terminator2/1  "<Torque_Command>"
  Bus Selector/4 -> Terminator3/1  "<Rotation_Direction>"
  Bus Creator2/1 -> Bus Creator1/2  "EM_Messages_Rhinehart"
  Bus Selector/5 -> Terminator1/1  "<BAS_Speed_Request>"
  Bus Selector/6 -> Bus Creator3/3  "<BAS_Mode_Request>"
  Bus Creator3/1 -> Bus Creator1/3  "BAS_SoftECU_Receive"
  Bus Selector/7 -> Terminator/1  "<ICE_Torque_Request_Nm>"
  Bus Selector/10 -> Bus Creator1/5  "<Trans_Receive>"
  ICE2/1 -> Bus Creator3/1  "BAS_Torque_Request_Nm"
  ICE3/1 -> Bus Creator2/2  "Torque_Command"
  ICE4/1 -> Bus Creator2/3  "Rotation_Direction"
  Bus Selector/11 -> Bus Creator1/6  "<Supervisory>"
  ICE5/1 -> Bus Creator3/2  "BAS_Speed_Request"
  Bus Creator4/1 -> Bus Creator1/4  "Engine_Messages"
  Bus Selector/8 -> Bus Creator4/2  "<Engine_On>"
  Bus Selector/9 -> Bus Creator4/3  "<Engine_Run>"
  ICE6/1 -> Bus Creator4/1  "ICE_Torque_Request_Nm"

== system EcoSIM3_P2_C2/Supervisory Controller/PRNDL/Park ==
  Treq : Inport
  Enable : EnablePort
  Bus Creator1 : BusCreator  Inputs=6
  Bus Creator2 : BusCreator  Inputs=3
  Bus Creator3 : BusCreator  Inputs=3
  Bus Creator4 : BusCreator  Inputs=3
  Bus Selector : BusSelector  OutputSignals=ESS_Signals_A123,EM_Messages_Rhinehart.Inverter_Enable,EM_Messages_Rhinehart.Torque_Command,EM_Messages_Rhinehart.Rotation_Direction,BAS_SoftECU_Receive.BAS_Torque_Request_Nm,BAS_SoftECU_Receive.BAS_Mode_Request,ICE_Request.ICE_Torque_Request_Nm,ICE_Request.Engine_On,ICE_Request.Engine_Run,Trans_Receive,Supervisory
  ICE{1..5} (5 alike) : Constant  Value=0
  Terminator{1..4} (4 alike) : Terminator
  HSC_Out : Outport
  wires:
  Bus Creator1/1 -> HSC_Out/1  "HSC_Out"
  Treq/1 -> Bus Selector/1
  Bus Selector/1 -> Bus Creator1/1  "<ESS_Signals_A123>"
  Bus Selector/2 -> Bus Creator2/1  "<Inverter_Enable>"
  Bus Selector/3 -> Terminator2/1  "<Torque_Command>"
  Bus Selector/4 -> Terminator3/1  "<Rotation_Direction>"
  Bus Creator2/1 -> Bus Creator1/2  "EM_Messages_Rhinehart"
  Bus Selector/5 -> Terminator1/1  "<BAS_Torque_Request_Nm>"
  Bus Selector/6 -> Bus Creator3/3  "<BAS_Mode_Request>"
  Bus Creator3/1 -> Bus Creator1/3  "BAS_SoftECU_Receive"
  Bus Selector/7 -> Terminator4/1  "<ICE_Torque_Request_Nm>"
  Bus Selector/10 -> Bus Creator1/5  "<Trans_Receive>"
  Bus Creator4/1 -> Bus Creator1/4  "Engine_Messages"
  ICE2/1 -> Bus Creator3/1  "BAS_Torque_Request_Nm"
  ICE3/1 -> Bus Creator2/2  "Torque_Command"
  ICE4/1 -> Bus Creator2/3  "Rotation_Direction"
  Bus Selector/11 -> Bus Creator1/6  "<Supervisory>"
  ICE5/1 -> Bus Creator3/2  "BAS_Speed_Request"
  Bus Selector/8 -> Bus Creator4/2  "<Engine_On>"
  Bus Selector/9 -> Bus Creator4/3  "<Engine_Run>"
  ICE1/1 -> Bus Creator4/1  "ICE_Torque_Request_Nm"

== system EcoSIM3_P2_C2/Supervisory Controller/PRNDL/Reverse ==
  Treq : Inport
  Enable : EnablePort
  Bus Creator : BusCreator  Inputs=6
  Bus Creator1 : BusCreator  Inputs=3
  Bus Creator2 : BusCreator  Inputs=3
  Bus Creator4 : BusCreator  Inputs=3
  Bus Selector : BusSelector  OutputSignals=ESS_Signals_A123,EM_Messages_Rhinehart.Inverter_Enable,EM_Messages_Rhinehart.Torque_Command,EM_Messages_Rhinehart.Rotation_Direction,BAS_SoftECU_Receive.BAS_Torque_Request_Nm,BAS_SoftECU_Receive.BAS_Mode_Request,ICE_Request.ICE_Torque_Request_Nm,ICE_Request.Engine_On,ICE_Request.Engine_Run,Trans_Receive,Supervisory
  Check BAS Limits : Subsystem
  Check EM Limits : Subsystem
  Ensure Desired Rotation Direction : Subsystem
  ICE5 : Constant  Value=0
  "HSC_Out " : Outport
  wires:
  Bus Creator/1 -> "HSC_Out "/1  "HSC_Out"
  Treq/1 -> Bus Selector/1
  Bus Selector/1 -> Bus Creator/1  "<ESS_Signals_A123>"
  Bus Selector/2 -> Bus Creator1/1  "<Inverter_Enable>"
  Bus Selector/3 -> Check EM Limits/1(In1)  "<Torque_Command>"
  Bus Selector/4 -> Bus Creator1/3  "<Rotation_Direction>"
  Bus Creator1/1 -> Bus Creator/2  "EM_Messages_Rhinehart"
  Bus Selector/5 -> Check BAS Limits/1(In1)  "<BAS_Torque_Request_Nm>"
  Bus Selector/6 -> Bus Creator2/3  "<BAS_Mode_Request>"
  Bus Creator2/1 -> Bus Creator/3  "BAS_SoftECU_Receive"
  Bus Selector/10 -> Bus Creator/5  "<Trans_Receive>"
  Check BAS Limits/1(Out1) -> Bus Creator2/1  "BAS_Torque_Request_Nm"
  Check EM Limits/1(Out1) -> Bus Creator1/2  "Torque_Command"
  Bus Selector/11 -> Bus Creator/6  "<Supervisory>"
  ICE5/1 -> Bus Creator2/2  "BAS_Speed_Request"
  Bus Creator4/1 -> Bus Creator/4  "Engine_Messages"
  Bus Selector/8 -> Bus Creator4/2  "<Engine_On>"
  Bus Selector/9 -> Bus Creator4/3  "<Engine_Run>"
  Bus Selector/7 -> Bus Creator4/1  "<ICE_Torque_Request_Nm>"

== system EcoSIM3_P2_C2/Supervisory Controller/Simple Fault Detection/CAN Communication Failures  ==
  In1 : Inport
  Out1 : Outport
  wires:
  In1/1 -> Out1/1

== system EcoSIM3_P2_C2/Supervisory Controller/Supervisory_IO/From_Goto ==
  Bus Creator : BusCreator  Inputs=7
  Bus Creator1 : BusCreator  Inputs=1
  Bus Selector1 : BusSelector  OutputSignals=GM_Transmit,ESS_Transmit,EM_Transmit,ICE_Transmit,Clutch_Transmission_SoftECU_Transmit,BAS_Transmit
  tag scope: From_Supervisory=global, From_Vehicle=global
  wires:
  Bus Creator/1 -> [From_Vehicle]
  [From_ECUs] -> Bus Selector1/1
  Bus Selector1/2 -> Bus Creator/3  "<ESS_Transmit>"
  Bus Selector1/3 -> Bus Creator/4  "<EM_Transmit>"
  Bus Selector1/4 -> Bus Creator/5  "<ICE_Transmit>"
  Bus Selector1/5 -> Bus Creator/6  "<Clutch_Transmission_SoftECU_Transmit>"
  Bus Selector1/6 -> Bus Creator/7  "<BAS_Transmit>"
  [From_GCM] -> Bus Creator/1
  [To_Vehicle] -> Bus Creator1/1
  Bus Creator1/1 -> [From_Supervisory]
  Bus Selector1/1 -> Bus Creator/2  "<GM_Transmit>"

== system EcoSIM3_P2_C2/Supervisory Controller/Supervisory_IO/VNT Kvaser ==
  CAN Rx : Subsystem
  CAN Tx : Subsystem
  Electrical Rx : Subsystem
  Electrical Tx : Subsystem
  Spine : Subsystem
  wires:
  Electrical Rx/1(Electrical_Rx) -> Spine/1(Electrical Rx)
  CAN Rx/1(CAN_Rx) -> Spine/2(CAN Rx)
  Spine/1(ElectricalTx) -> Electrical Tx/1(Electrical Tx)
  Spine/2(CANTx) -> CAN Tx/1(CAN Tx)

== system EcoSIM3_P2_C2/Supervisory Controller/Supervisory_IO/VNT Vector ==
  CAN Rx : Subsystem
  CAN Tx : Subsystem
  Electrical Rx : Subsystem
  Electrical Tx : Subsystem
  Spine : Subsystem
  wires:
  Electrical Rx/1(Electrical_Rx) -> Spine/1(Electrical Rx)
  CAN Rx/1(CAN_Rx) -> Spine/2(CAN Rx)
  Spine/1(ElectricalTx) -> Electrical Tx/1(Electrical Tx)
  Spine/2(CANTx) -> CAN Tx/1(CAN Tx)

== system EcoSIM3_P2_C2/GCM/GCM_IO/VNT Kvaser/CAN Rx ==
  note: This is a digital signal. So use from goto.
  Ground : Ground
  CAN : Outport
  wires:
  Ground/1 -> CAN/1

== system EcoSIM3_P2_C2/GCM/GCM_IO/VNT Kvaser/CAN Tx ==
  CAN : Inport
  Bus Selector : BusSelector  OutputSignals=charge_mode_request
  CAN Pack6 : canmsglib/CAN Pack  CANdbFile=C:\Users\EcoCAR_HIL\Documents\Khanna\EcoSIM3_P1_0_PHEV_TCU\Final_DBC\EcoCAR3_Controls_Development.dbc  MsgList=GCM_Transmit_MSG096  MsgName=GCM_Transmit_MSG096  MsgIDType=Standard (11-bit identifier)  MsgIdentifier=96  MsgLength=1  SignalInfo=charge_mode_request$7$1$2$2$1$0$1$0$0$1$#  NSignals=1  StartBits=str2num('[int32(7)]')  SignalSizes=str2num('[int32(1)]')  ByteOrders=str2num('[int32(2)]')  DataTypes=str2num('[int32(2)]')  MultiplexTypes=str2num('[int32(1)]')  MultiplexValues=str2num('[double(0)]')  Factors=str2num('[double(1)]')  Offsets=str2num('[double(0)]')  Minimums=str2num('[double(0)]')  Maximums=str2num('[double(1)]')  Remote=off
      settings: DataFormat=CANdb specified signals
  CAN Transmit6 : canlib/CAN Transmit  BlockHandle=371.0007  DeviceMenu=Kvaser Virtual 1 (Channel 1)  Device=Kvaser Virtual 1 (Channel 1)  ObjConstructor=canChannel('Kvaser', 'Virtual 1', 1)  EnablePeriodicTransmit=off  MessagePeriod=1.000
  Rate Transition : RateTransition
  wires:
  CAN Pack6/1 -> CAN Transmit6/1
  CAN/1 -> Bus Selector/1
  Bus Selector/1 -> Rate Transition/1  "<charge_mode_request>"
  Rate Transition/1 -> CAN Pack6/1

== system EcoSIM3_P2_C2/GCM/GCM_IO/VNT Kvaser/Electrical Rx ==
  Bus Creator{,1..3} (4 alike) : BusCreator  Inputs=1
  Bus Creator5 : BusCreator  Inputs=2
  Bus Selector : BusSelector  OutputSignals=GM_Electrical_Out.Key_State,Brusa_Electrical_Out.GCM_Wakeup_charge
  Electrical : Outport
  wires:
  [VNT_Electrical_From_SoftECU] -> Bus Selector/1
  Bus Creator5/1 -> Electrical/1
  Bus Creator3/1 -> Bus Creator5/2  "Brusa_Transmit"
  Bus Creator1/1 -> Bus Creator5/1  "GM_Transmit"
  Bus Creator2/1 -> Bus Creator3/1  "Brusa_Electrical_Out"
  Bus Creator/1 -> Bus Creator1/1  "GM_Electrical_Out"
  Bus Selector/1 -> Bus Creator/1  "<Key_State>"
  Bus Selector/2 -> Bus Creator2/1  "<GCM_Wakeup_charge>"

== system EcoSIM3_P2_C2/GCM/GCM_IO/VNT Kvaser/Electrical Tx ==
  Electrical : Inport
  tag scope: VNT_Electrical_FromGCM=global
  wires:
  Electrical/1 -> [VNT_Electrical_FromGCM]

== system EcoSIM3_P2_C2/GCM/GCM_IO/VNT Kvaser/Spine ==
  note: This is a digital signal. So use from goto.
  Electrical Rx : Inport
  CAN Rx : Inport  Port=2
  Bus Selector : BusSelector  OutputSignals=GCM_Electrical_Out,GCM_CAN_Out
  Terminator : Terminator
  Electrical Tx : Outport
  CAN Tx : Outport  Port=2
  tag scope: GCM_from_CAN=global
  wires:
  [GCM_To_CAN] -> Bus Selector/1
  Electrical Rx/1 -> [GCM_from_CAN]
  CAN Rx/1 -> Terminator/1
  Bus Selector/1 -> Electrical Tx/1  "<GCM_Electrical_Out>"
  Bus Selector/2 -> CAN Tx/1  "<GCM_CAN_Out>"

== system EcoSIM3_P2_C2/GCM/GCM_IO/VNT Vector/CAN Rx ==
  note: This is a digital signal. So use from goto.
  Ground : Ground
  CAN : Outport
  wires:
  Ground/1 -> CAN/1

== system EcoSIM3_P2_C2/GCM/GCM_IO/VNT Vector/CAN Tx ==
  CAN : Inport
  Bus Selector : BusSelector  OutputSignals=charge_mode_request
  CAN Pack6 : canmsglib/CAN Pack  CANdbFile=C:\Users\EcoCAR_HIL\Documents\Khanna\EcoSIM3_P1_0_PHEV_TCU\Final_DBC\EcoCAR3_Controls_Development.dbc  MsgList=GCM_Transmit_MSG096  MsgName=GCM_Transmit_MSG096  MsgIDType=Standard (11-bit identifier)  MsgIdentifier=96  MsgLength=1  SignalInfo=charge_mode_request$7$1$2$2$1$0$1$0$0$1$#  NSignals=1  StartBits=str2num('[int32(7)]')  SignalSizes=str2num('[int32(1)]')  ByteOrders=str2num('[int32(2)]')  DataTypes=str2num('[int32(2)]')  MultiplexTypes=str2num('[int32(1)]')  MultiplexValues=str2num('[double(0)]')  Factors=str2num('[double(1)]')  Offsets=str2num('[double(0)]')  Minimums=str2num('[double(0)]')  Maximums=str2num('[double(1)]')  Remote=off
      settings: DataFormat=CANdb specified signals
  CAN Transmit6 : canlib/CAN Transmit  BlockHandle=9459.0199  DeviceMenu=Vector Virtual 1 (Channel 1)  Device=Vector Virtual 1 (Channel 1)  ObjConstructor=canChannel('Vector', 'Virtual 1', 1)  EnablePeriodicTransmit=off  MessagePeriod=1.000
  Rate Transition : RateTransition
  wires:
  CAN Pack6/1 -> CAN Transmit6/1
  CAN/1 -> Bus Selector/1
  Bus Selector/1 -> Rate Transition/1  "<charge_mode_request>"
  Rate Transition/1 -> CAN Pack6/1

== system EcoSIM3_P2_C2/GCM/GCM_IO/VNT Vector/Electrical Rx ==
  Bus Creator{,1..3} (4 alike) : BusCreator  Inputs=1
  Bus Creator5 : BusCreator  Inputs=2
  Bus Selector : BusSelector  OutputSignals=GM_Electrical_Out.Key_State,Brusa_Electrical_Out.GCM_Wakeup_charge
  Electrical : Outport
  wires:
  [VNT_Electrical_From_SoftECU] -> Bus Selector/1
  Bus Creator5/1 -> Electrical/1
  Bus Creator3/1 -> Bus Creator5/2  "Brusa_Transmit"
  Bus Creator1/1 -> Bus Creator5/1  "GM_Transmit"
  Bus Creator2/1 -> Bus Creator3/1  "Brusa_Electrical_Out"
  Bus Creator/1 -> Bus Creator1/1  "GM_Electrical_Out"
  Bus Selector/1 -> Bus Creator/1  "<Key_State>"
  Bus Selector/2 -> Bus Creator2/1  "<GCM_Wakeup_charge>"

== system EcoSIM3_P2_C2/GCM/GCM_IO/VNT Vector/Electrical Tx ==
  Electrical : Inport
  tag scope: VNT_Electrical_FromGCM=global
  wires:
  Electrical/1 -> [VNT_Electrical_FromGCM]

== system EcoSIM3_P2_C2/GCM/GCM_IO/VNT Vector/Spine ==
  note: This is a digital signal. So use from goto.
  Electrical Rx : Inport
  CAN Rx : Inport  Port=2
  Bus Selector : BusSelector  OutputSignals=GCM_Electrical_Out,GCM_CAN_Out
  Terminator : Terminator
  Electrical Tx : Outport
  CAN Tx : Outport  Port=2
  tag scope: GCM_from_CAN=global
  wires:
  [GCM_To_CAN] -> Bus Selector/1
  Electrical Rx/1 -> [GCM_from_CAN]
  CAN Rx/1 -> Terminator/1
  Bus Selector/1 -> Electrical Tx/1  "<GCM_Electrical_Out>"
  Bus Selector/2 -> CAN Tx/1  "<GCM_CAN_Out>"

== system EcoSIM3_P2_C2/Powertrain/Accessories/The Corrupter/Enabled Subsystem ==
  In1 : Inport
  In2 : Inport  Port=2
  Enable : EnablePort
  Integrator : Integrator  InitialCondition=100
  Product5 : Product  Inputs=*/  RndMeth=Zero
  Out1 : Outport
  wires:
  Integrator/1 -> Out1/1
  In2/1 -> Product5/2
  In1/1 -> Product5/1
  Product5/1 -> Integrator/1

== system EcoSIM3_P2_C2/Powertrain/Accessories/The Corrupter/Switch Logic ==
  NonCorrupted : Inport
  Corrupted : Inport  Port=2
  Logic : Inport  Port=3
  Switch : Switch  Criteria=u2 > Threshold
  Signal Out : Outport
  wires:
  Switch/1 -> Signal Out/1
  Logic/1 -> Switch/2
  NonCorrupted/1 -> Switch/3
  Corrupted/1 -> Switch/1
